simulink model "PUMA560robot_simulink"  (R2023a)
settings: Solver=ode4  StartTime=0.0  StopTime=10  FixedStep=0.001  RelTol=1e-3
values from neighbouring files (symbols this model uses):
  A = [zeros(3,3),eye(3,3) ... (first row only)    [main_PUMA560robot.m]
  B = [0   0   0 ... (first row only)    [main_PUMA560robot.m]
  d = norm(ep_-R_)    [main_PUMA560robot.m]
  Fcdirec = [1,100,1,0.001,           0.5,100,1,0.001,           1,300,1,0.3,           1,200,1,0.1,           2.5,100,2,0.01,           0.5,200,1,0.02]    [main_PUMA560robot.m]
  Kall = cat(1,Kall,K_)    [main_PUMA560robot.m]
  m = size(B',1)    [main_PUMA560robot.m]
  nK0 = 1    [main_PUMA560robot.m]
  Pall = cat(1,Pall,P_)    [main_PUMA560robot.m]
  R0q = Rall(1:3,1:3)    [main_PUMA560robot.m]
  rho = zeros(N,1)    [main_PUMA560robot.m]
  rhospan = linspace(0,1043,100000)    [main_PUMA560robot.m]
  umax = [97.8 136.4 89.4]    [main_PUMA560robot.m]
  x0 = 10/sqrt(6)* [1;1;1;1;1;1]    [main_PUMA560robot.m]
undefined symbols (not defined in the file or in its folder): Kb, Pb, Pcq
settings Model: Creator=shuyuanfan  LastModifiedBy=fansh

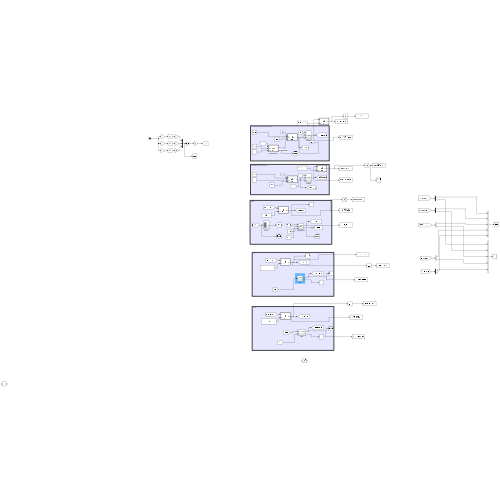
[thumbnail: Simulink's stored preview of the top-level diagram]
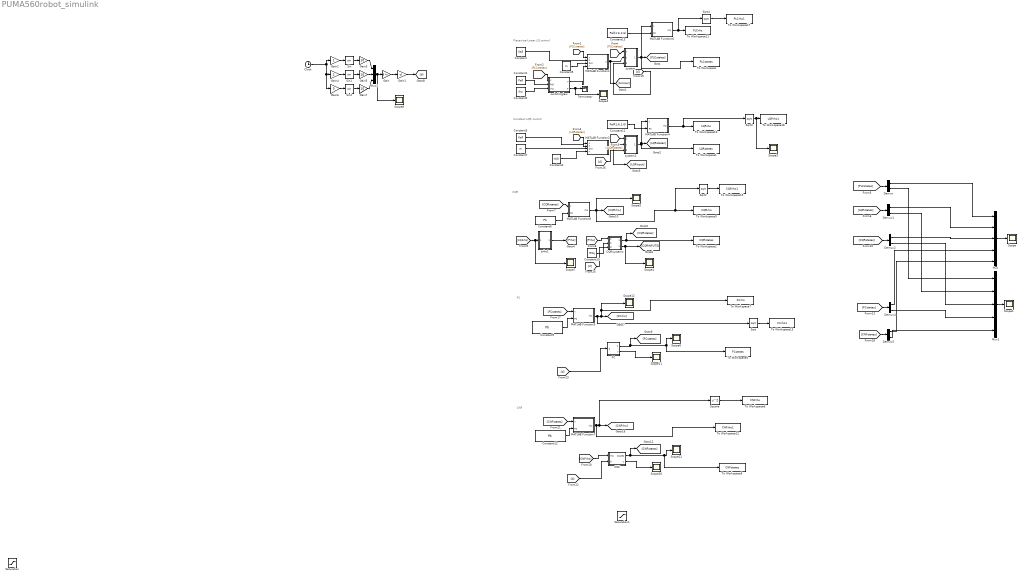
== system PUMA560robot_simulink ==
  note: CQR
  note: Piecewise-Linear LQ control
  note: Constant LQR control
  note: FC
  note: CNF
  CNF : Subsystem
  CQRsystems : Subsystem
  Clock : Clock
  Constant : Constant  Value=Kall
  Constant1 : Constant  Value=Pall
  Constant10 : Constant  Value=R0q
  Constant11 : Constant  Value=Pall(1:6,1:6)
  Constant12 : Constant  Value=Pb
  Constant13 : Constant  Value=Pall(1:6,1:6)
  Constant2 : Constant  Value=rho
  Constant3 : Constant  Value=Kall
  Constant4 : Constant  Value=nK0
  Constant5 : Constant  Value=m
  Constant6 : Constant  Value=Pb
  Constant7 : Constant  Value=m
  Constant9 : Constant  Value=Pb
  Demux{,1..2,4..5} (5 alike) : Demux  Outputs=2
  FC : Subsystem
  Gain : Gain  Gain=B  Multiplication=Matrix(K*u)
  Gain1 : Gain  Gain=d
  Gain2 : Gain
  Gain3 : Gain  Gain=10
  Gain4 : Gain  Gain=2
  Gain5 : Gain  Gain=10
  Gain6 : Gain  Gain=3
  Gain7 : Gain  Gain=10
  MATLAB Function1 : MATLAB Function  TreatAsAtomicUnit=on
  MATLAB Function2 : MATLAB Function  TreatAsAtomicUnit=on
  MATLAB Function3 : MATLAB Function  TreatAsAtomicUnit=on
  MATLAB Function4 : MATLAB Function  TreatAsAtomicUnit=on
  MATLAB Function6 : MATLAB Function  TreatAsAtomicUnit=on
  MATLAB Function7 : MATLAB Function  TreatAsAtomicUnit=on
  MATLAB Function8 : MATLAB Function  TreatAsAtomicUnit=on
  Mux : Mux  Inputs=5
  Mux1 : Mux  Inputs=5
  Mux2 : Mux  Inputs=3
  Saturation : Saturate  UpperLimit=umax'  LowerLimit=-umax'
  Saturation1 : Saturate  UpperLimit=umax'  LowerLimit=-umax'
  Scope{,1..8,11..12,20,22} (13 alike) : Scope
  Sin : Trigonometry
  Sin1 : Trigonometry
  Sin2 : Trigonometry
  Sqrt{,2..4} (4 alike) : Sqrt
  Square : Math  Operator=square
  Terminator : Terminator
  To Workspace : ToWorkspace  VariableName=PLCstates  SaveFormat=Timeseries  SampleTime=-1
  To Workspace1 : ToWorkspace  VariableName=LQRstates  SaveFormat=Timeseries  SampleTime=-1
  To Workspace10 : ToWorkspace  VariableName=LQRrho  SaveFormat=Timeseries  SampleTime=-1
  To Workspace11 : ToWorkspace  VariableName=PLCrho  SaveFormat=Timeseries  SampleTime=-1
  To Workspace12 : ToWorkspace  VariableName=CNFrho1  SaveFormat=Timeseries  SampleTime=-1
  To Workspace13 : ToWorkspace  VariableName=FCrho1  SaveFormat=Timeseries  SampleTime=-1
  To Workspace15 : ToWorkspace  VariableName=CQRrho1  SaveFormat=Timeseries  SampleTime=-1
  To Workspace16 : ToWorkspace  VariableName=LQRrho1  SaveFormat=Timeseries  SampleTime=-1
  To Workspace17 : ToWorkspace  VariableName=PLCrho1  SaveFormat=Timeseries  SampleTime=-1
  To Workspace2 : ToWorkspace  VariableName=CQRstates  SaveFormat=Timeseries  SampleTime=-1
  To Workspace4 : ToWorkspace  VariableName=FCstates  SaveFormat=Timeseries  SampleTime=-1
  To Workspace5 : ToWorkspace  VariableName=CNFstates  SaveFormat=Timeseries  SampleTime=-1
  To Workspace6 : ToWorkspace  VariableName=CNFrho  SaveFormat=Timeseries  SampleTime=-1
  To Workspace7 : ToWorkspace  VariableName=FCrho  SaveFormat=Timeseries  SampleTime=-1
  To Workspace9 : ToWorkspace  VariableName=CQRrho  SaveFormat=Timeseries  SampleTime=-1
  prho1 : Subsystem
  switchinglaw : MATLAB Function  TreatAsAtomicUnit=on
  system : Subsystem
  system2 : Subsystem
  wires:
  Constant/1 -> MATLAB Function1/2(K)
  Constant1/1 -> switchinglaw/2(Pall)
  Constant2/1 -> switchinglaw/3(rho)
  system/1(states) -> MATLAB Function6/1(x), To Workspace/1, [PLCstates]
  [PLCstates] -> system/1(x)
  [PLCstates] -> MATLAB Function1/1(x)
  [PLCstates] -> switchinglaw/1(x)
  MATLAB Function1/1(u) -> system/2(u), [PLCinput]
  MATLAB Function2/1(u) -> system2/2(u), [LQRinput]
  Constant3/1 -> MATLAB Function2/2(K)
  Constant4/1 -> MATLAB Function2/4(n)
  system2/1(states) -> MATLAB Function4/1(x), [LQRstates], To Workspace1/1
  [LQRstates] -> MATLAB Function2/1(x)
  Constant7/1 -> MATLAB Function2/3(dim)
  [LQRstates] -> system2/1(x)
  switchinglaw/1(n) -> MATLAB Function1/4(n)
  Constant5/1 -> MATLAB Function1/3(dim)
  switchinglaw/2(F) -> Scope2/1, Terminator/1
  [CQRstates] -> MATLAB Function8/1(x)
  [CQRrho] -> Scope7/1, prho1/1(In1)
  MATLAB Function8/1(rho) -> Scope5/1, Sqrt2/1, To Workspace9/1, [CQRrho]
  Constant6/1 -> MATLAB Function8/2(P0)
  CQRsystems/2(u) -> Scope4/1, [CQRINPUTS]
  CQRsystems/1(states) -> To Workspace2/1, [CQRstates]
  [Prho] -> CQRsystems/1(p)
  Constant10/1 -> CQRsystems/2(paraR)
  prho1/1(Out1) -> [Prho]
  FC/2(u) -> Scope11/1
  FC/1(states) -> Scope6/1, To Workspace4/1, [FCstates]
  [FCstates] -> MATLAB Function3/1(x)
  Constant9/1 -> MATLAB Function3/2(P0)
  MATLAB Function3/1(rho) -> Sqrt/1, To Workspace7/1, Scope12/1, [FCrho]
  [CNFstates] -> MATLAB Function7/1(x)
  CNF/2(u) -> Scope20/1
  [CNFrho] -> CNF/1(rho)
  Constant12/1 -> MATLAB Function7/2(P0)
  MATLAB Function7/1(rho) -> To Workspace12/1, Square/1, [CNFrho]
  CNF/1(states) -> To Workspace5/1, Scope22/1, [CNFstates]
  [PLCstates] -> Demux/1
  [LQRstates] -> Demux1/1
  [CQRstates] -> Demux2/1
  [FCstates] -> Demux4/1
  [CNFstates] -> Demux5/1
  Demux/1 -> Mux/1
  Demux1/1 -> Mux/2
  Demux2/1 -> Mux/3
  Demux4/1 -> Mux/4
  Demux5/1 -> Mux/5
  Demux/2 -> Mux1/1
  Demux1/2 -> Mux1/2
  Demux2/2 -> Mux1/3
  Demux4/2 -> Mux1/4
  Demux5/2 -> Mux1/5
  Mux/1 -> Scope/1
  Mux1/1 -> Scope1/1
  Square/1 -> To Workspace6/1
  MATLAB Function4/1(rho) -> Sqrt3/1, To Workspace10/1
  Constant11/1 -> MATLAB Function4/2(P0)
  Constant13/1 -> MATLAB Function6/2(P0)
  MATLAB Function6/1(rho) -> Sqrt4/1, To Workspace11/1
  Sqrt/1 -> To Workspace13/1
  Sqrt2/1 -> To Workspace15/1
  Sqrt3/1 -> Scope3/1, To Workspace16/1
  Sqrt4/1 -> To Workspace17/1
  Gain1/1 -> [d]
  [d] -> system/3(d)
  [d] -> system2/3(d)
  [d] -> CQRsystems/3(d)
  [d] -> FC/1(d)
  [d] -> CNF/2(d)
  Gain/1 -> Gain1/1
  Gain2/1 -> Sin/1
  Sin/1 -> Gain3/1
  Sin1/1 -> Gain5/1
  Gain4/1 -> Sin1/1
  Clock/1 -> Gain6/1, Gain4/1, Gain2/1
  Sin2/1 -> Gain7/1
  Gain6/1 -> Sin2/1
  Gain5/1 -> Mux2/2
  Gain3/1 -> Mux2/1
  Gain7/1 -> Mux2/3
  Mux2/1 -> Scope8/1, Gain/1

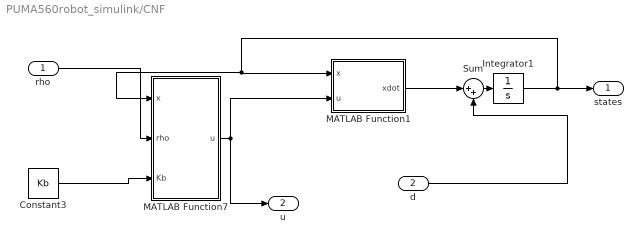
== system PUMA560robot_simulink/CNF ==
  rho : Inport
  d : Inport  Port=2
  Constant3 : Constant  Value=Kb
  Integrator1 : Integrator  InitialCondition=x0
  MATLAB Function1 : MATLAB Function  TreatAsAtomicUnit=on
  MATLAB Function7 : MATLAB Function  TreatAsAtomicUnit=on
  Sum : Sum  Inputs=|++
  states : Outport
  u : Outport  Port=2
  wires:
  Integrator1/1 -> states/1, MATLAB Function1/1(x), MATLAB Function7/1(x)
  MATLAB Function1/1(xdot) -> Sum/1
  Sum/1 -> Integrator1/1
  d/1 -> Sum/2
  rho/1 -> MATLAB Function7/2(rho)
  Constant3/1 -> MATLAB Function7/3(Kb)
  MATLAB Function7/1(u) -> MATLAB Function1/2(u), u/1

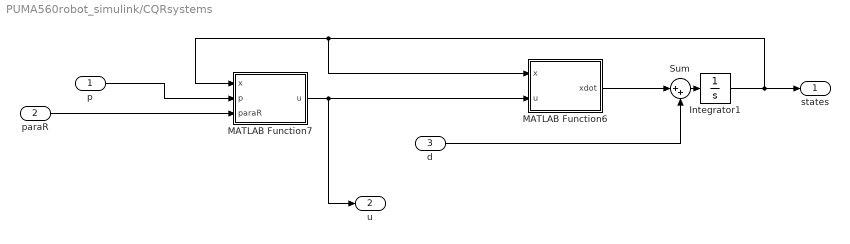
== system PUMA560robot_simulink/CQRsystems ==
  p : Inport
  paraR : Inport  Port=2
  d : Inport  Port=3
  Integrator1 : Integrator  InitialCondition=x0
  MATLAB Function6 : MATLAB Function  TreatAsAtomicUnit=on
  MATLAB Function7 : MATLAB Function  TreatAsAtomicUnit=on
  Sum : Sum  Inputs=|++
  states : Outport
  u : Outport  Port=2
  wires:
  Integrator1/1 -> states/1, MATLAB Function6/1(x), MATLAB Function7/1(x)
  MATLAB Function6/1(xdot) -> Sum/1
  paraR/1 -> MATLAB Function7/3(paraR)
  p/1 -> MATLAB Function7/2(p)
  Sum/1 -> Integrator1/1
  d/1 -> Sum/2
  MATLAB Function7/1(u) -> MATLAB Function6/2(u), u/1

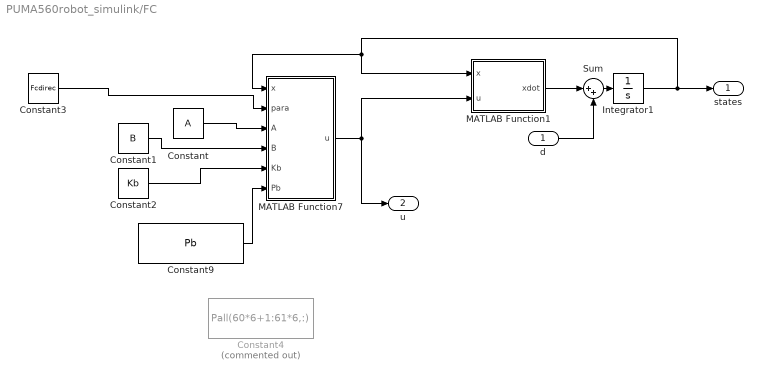
== system PUMA560robot_simulink/FC ==
  d : Inport
  Constant : Constant  Value=A
  Constant1 : Constant  Value=B
  Constant2 : Constant  Value=Kb
  Constant3 : Constant  Value=Fcdirec
  Constant4 : Constant  Commented=on  Value=Pall(60*6+1:61*6,:)
  Constant9 : Constant  Value=Pb
  Integrator1 : Integrator  InitialCondition=x0
  MATLAB Function1 : MATLAB Function  TreatAsAtomicUnit=on
  MATLAB Function7 : MATLAB Function  TreatAsAtomicUnit=on
  Sum : Sum  Inputs=|++
  states : Outport
  u : Outport  Port=2
  wires:
  Integrator1/1 -> states/1, MATLAB Function1/1(x), MATLAB Function7/1(x)
  MATLAB Function1/1(xdot) -> Sum/1
  Sum/1 -> Integrator1/1
  Constant/1 -> MATLAB Function7/3(A)
  Constant1/1 -> MATLAB Function7/4(B)
  Constant2/1 -> MATLAB Function7/5(Kb)
  Constant9/1 -> MATLAB Function7/6(Pb)
  d/1 -> Sum/2
  MATLAB Function7/1(u) -> MATLAB Function1/2(u), u/1
  Constant3/1 -> MATLAB Function7/2(para)

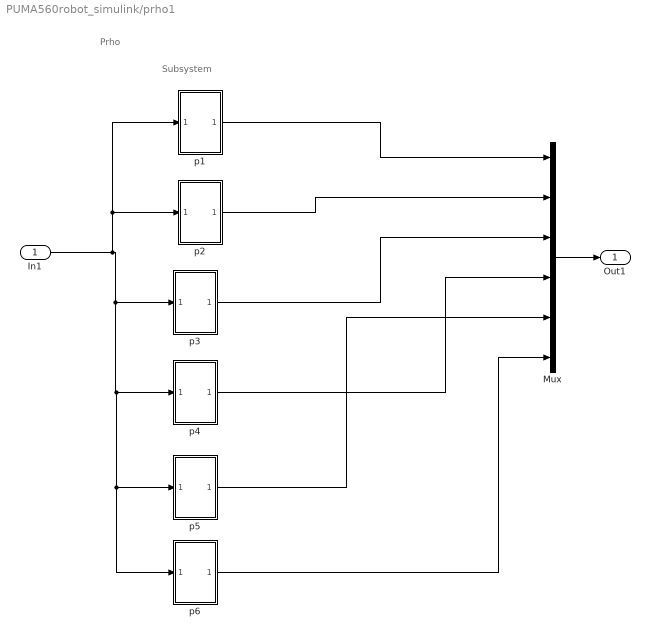
== system PUMA560robot_simulink/prho1 ==
  note: Prho
  note: Subsystem
  In1 : Inport
  Mux : Mux  Inputs=6
  p1 : Subsystem
  p2 : Subsystem
  p3 : Subsystem
  p4 : Subsystem
  p5 : Subsystem
  p6 : Subsystem
  Out1 : Outport
  wires:
  p4/1(Out1) -> Mux/4
  In1/1 -> p6/1(In1), p5/1(In1), p4/1(In1), p3/1(In1), p2/1(In1), p1/1(In1)
  Mux/1 -> Out1/1
  p1/1(Out1) -> Mux/1
  p3/1(Out1) -> Mux/3
  p2/1(Out1) -> Mux/2
  p5/1(Out1) -> Mux/5
  p6/1(Out1) -> Mux/6

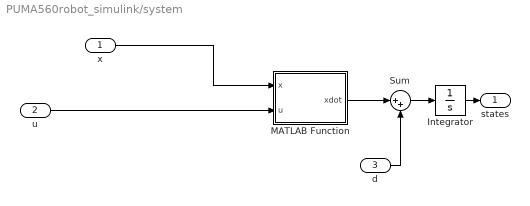
== system PUMA560robot_simulink/system ==
  x : Inport
  u : Inport  Port=2
  d : Inport  Port=3
  Integrator : Integrator  InitialCondition=x0
  MATLAB Function : MATLAB Function  TreatAsAtomicUnit=on
  Sum : Sum  Inputs=|++
  states : Outport
  wires:
  x/1 -> MATLAB Function/1(x)
  Integrator/1 -> states/1
  MATLAB Function/1(xdot) -> Sum/1
  Sum/1 -> Integrator/1
  d/1 -> Sum/2
  u/1 -> MATLAB Function/2(u)

== system PUMA560robot_simulink/system2 ==
  x : Inport
  u : Inport  Port=2
  d : Inport  Port=3
  Integrator : Integrator  InitialCondition=x0
  MATLAB Function : MATLAB Function  TreatAsAtomicUnit=on
  Sum : Sum  Inputs=|++
  states : Outport
  wires:
  x/1 -> MATLAB Function/1(x)
  Integrator/1 -> states/1
  MATLAB Function/1(xdot) -> Sum/1
  Sum/1 -> Integrator/1
  d/1 -> Sum/2
  u/1 -> MATLAB Function/2(u)

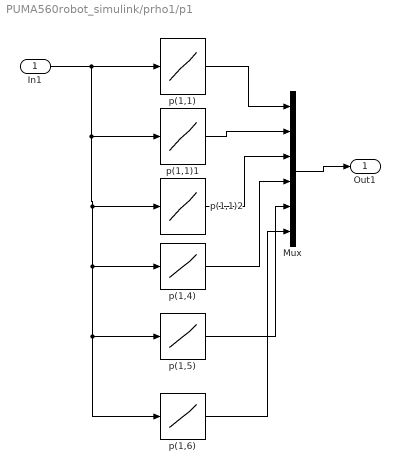
== system PUMA560robot_simulink/prho1/p1 ==
  In1 : Inport
  Mux : Mux  Inputs=6
  p(1,1) : Lookup_n-D  NumberOfTableDimensions=1  BreakpointsForDimension1=rhospan  Table=Pcq(:,1)  InterpMethod=Linear Lagrange  InternalRulePriority=Speed  RndMeth=Simplest
  p(1,1)1 : Lookup_n-D  NumberOfTableDimensions=1  BreakpointsForDimension1=rhospan  Table=Pcq(:,2)  InterpMethod=Linear Lagrange  InternalRulePriority=Speed  RndMeth=Simplest
  p(1,1)2 : Lookup_n-D  NumberOfTableDimensions=1  BreakpointsForDimension1=rhospan  Table=Pcq(:,3)  InterpMethod=Linear Lagrange  InternalRulePriority=Speed  RndMeth=Simplest
  p(1,4) : Lookup_n-D  NumberOfTableDimensions=1  BreakpointsForDimension1=rhospan  Table=Pcq(:,4)  InterpMethod=Linear Lagrange  InternalRulePriority=Speed  RndMeth=Simplest
  p(1,5) : Lookup_n-D  NumberOfTableDimensions=1  BreakpointsForDimension1=rhospan  Table=Pcq(:,5)  InterpMethod=Linear Lagrange  InternalRulePriority=Speed  RndMeth=Simplest
  p(1,6) : Lookup_n-D  NumberOfTableDimensions=1  BreakpointsForDimension1=rhospan  Table=Pcq(:,6)  InterpMethod=Linear Lagrange  InternalRulePriority=Speed  RndMeth=Simplest
  Out1 : Outport
  wires:
  p(1,1)1/1 -> Mux/2
  p(1,4)/1 -> Mux/4
  In1/1 -> p(1,1)1/1, p(1,1)2/1, p(1,6)/1, p(1,5)/1, p(1,4)/1, p(1,1)/1
  p(1,1)/1 -> Mux/1
  p(1,1)2/1 -> Mux/3
  Mux/1 -> Out1/1
  p(1,5)/1 -> Mux/5
  p(1,6)/1 -> Mux/6

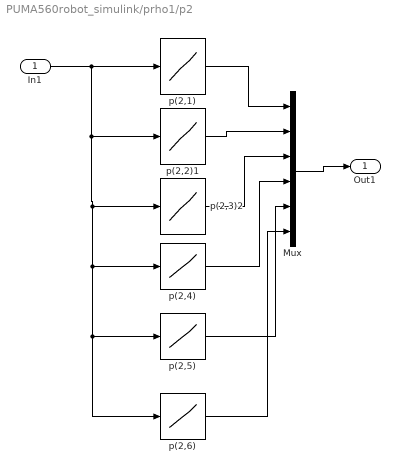
== system PUMA560robot_simulink/prho1/p2 ==
  In1 : Inport
  Mux : Mux  Inputs=6
  p(2,1) : Lookup_n-D  NumberOfTableDimensions=1  BreakpointsForDimension1=rhospan  Table=Pcq(:,7)  InterpMethod=Linear Lagrange  InternalRulePriority=Speed  RndMeth=Simplest
  p(2,2)1 : Lookup_n-D  NumberOfTableDimensions=1  BreakpointsForDimension1=rhospan  Table=Pcq(:,8)  InterpMethod=Linear Lagrange  InternalRulePriority=Speed  RndMeth=Simplest
  p(2,3)2 : Lookup_n-D  NumberOfTableDimensions=1  BreakpointsForDimension1=rhospan  Table=Pcq(:,9)  InterpMethod=Linear Lagrange  InternalRulePriority=Speed  RndMeth=Simplest
  p(2,4) : Lookup_n-D  NumberOfTableDimensions=1  BreakpointsForDimension1=rhospan  Table=Pcq(:,10)  InterpMethod=Linear Lagrange  InternalRulePriority=Speed  RndMeth=Simplest
  p(2,5) : Lookup_n-D  NumberOfTableDimensions=1  BreakpointsForDimension1=rhospan  Table=Pcq(:,11)  InterpMethod=Linear Lagrange  InternalRulePriority=Speed  RndMeth=Simplest
  p(2,6) : Lookup_n-D  NumberOfTableDimensions=1  BreakpointsForDimension1=rhospan  Table=Pcq(:,12)  InterpMethod=Linear Lagrange  InternalRulePriority=Speed  RndMeth=Simplest
  Out1 : Outport
  wires:
  p(2,2)1/1 -> Mux/2
  p(2,4)/1 -> Mux/4
  In1/1 -> p(2,2)1/1, p(2,3)2/1, p(2,6)/1, p(2,5)/1, p(2,4)/1, p(2,1)/1
  p(2,1)/1 -> Mux/1
  p(2,3)2/1 -> Mux/3
  Mux/1 -> Out1/1
  p(2,5)/1 -> Mux/5
  p(2,6)/1 -> Mux/6

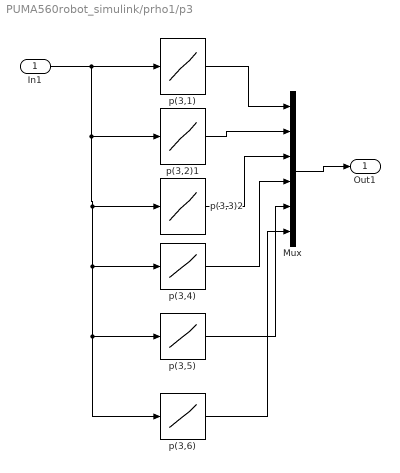
== system PUMA560robot_simulink/prho1/p3 ==
  In1 : Inport
  Mux : Mux  Inputs=6
  p(3,1) : Lookup_n-D  NumberOfTableDimensions=1  BreakpointsForDimension1=rhospan  Table=Pcq(:,13)  InterpMethod=Linear Lagrange  InternalRulePriority=Speed  RndMeth=Simplest
  p(3,2)1 : Lookup_n-D  NumberOfTableDimensions=1  BreakpointsForDimension1=rhospan  Table=Pcq(:,14)  InterpMethod=Linear Lagrange  InternalRulePriority=Speed  RndMeth=Simplest
  p(3,3)2 : Lookup_n-D  NumberOfTableDimensions=1  BreakpointsForDimension1=rhospan  Table=Pcq(:,15)  InterpMethod=Linear Lagrange  InternalRulePriority=Speed  RndMeth=Simplest
  p(3,4) : Lookup_n-D  NumberOfTableDimensions=1  BreakpointsForDimension1=rhospan  Table=Pcq(:,16)  InterpMethod=Linear Lagrange  InternalRulePriority=Speed  RndMeth=Simplest
  p(3,5) : Lookup_n-D  NumberOfTableDimensions=1  BreakpointsForDimension1=rhospan  Table=Pcq(:,17)  InterpMethod=Linear Lagrange  InternalRulePriority=Speed  RndMeth=Simplest
  p(3,6) : Lookup_n-D  NumberOfTableDimensions=1  BreakpointsForDimension1=rhospan  Table=Pcq(:,18)  InterpMethod=Linear Lagrange  InternalRulePriority=Speed  RndMeth=Simplest
  Out1 : Outport
  wires:
  p(3,2)1/1 -> Mux/2
  p(3,4)/1 -> Mux/4
  In1/1 -> p(3,2)1/1, p(3,3)2/1, p(3,6)/1, p(3,5)/1, p(3,4)/1, p(3,1)/1
  p(3,1)/1 -> Mux/1
  p(3,3)2/1 -> Mux/3
  Mux/1 -> Out1/1
  p(3,5)/1 -> Mux/5
  p(3,6)/1 -> Mux/6

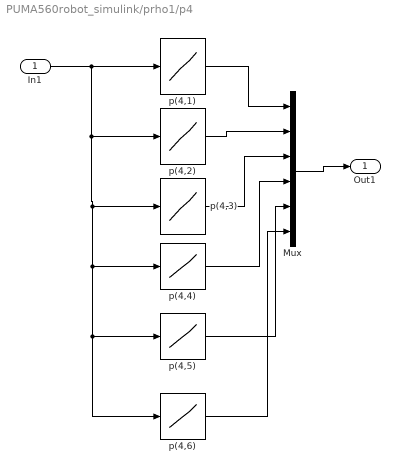
== system PUMA560robot_simulink/prho1/p4 ==
  In1 : Inport
  Mux : Mux  Inputs=6
  p(4,1) : Lookup_n-D  NumberOfTableDimensions=1  BreakpointsForDimension1=rhospan  Table=Pcq(:,19)  InterpMethod=Linear Lagrange  InternalRulePriority=Speed  RndMeth=Simplest
  p(4,2) : Lookup_n-D  NumberOfTableDimensions=1  BreakpointsForDimension1=rhospan  Table=Pcq(:,20)  InterpMethod=Linear Lagrange  InternalRulePriority=Speed  RndMeth=Simplest
  p(4,3) : Lookup_n-D  NumberOfTableDimensions=1  BreakpointsForDimension1=rhospan  Table=Pcq(:,21)  InterpMethod=Linear Lagrange  InternalRulePriority=Speed  RndMeth=Simplest
  p(4,4) : Lookup_n-D  NumberOfTableDimensions=1  BreakpointsForDimension1=rhospan  Table=Pcq(:,22)  InterpMethod=Linear Lagrange  InternalRulePriority=Speed  RndMeth=Simplest
  p(4,5) : Lookup_n-D  NumberOfTableDimensions=1  BreakpointsForDimension1=rhospan  Table=Pcq(:,23)  InterpMethod=Linear Lagrange  InternalRulePriority=Speed  RndMeth=Simplest
  p(4,6) : Lookup_n-D  NumberOfTableDimensions=1  BreakpointsForDimension1=rhospan  Table=Pcq(:,24)  InterpMethod=Linear Lagrange  InternalRulePriority=Speed  RndMeth=Simplest
  Out1 : Outport
  wires:
  p(4,2)/1 -> Mux/2
  p(4,4)/1 -> Mux/4
  In1/1 -> p(4,2)/1, p(4,3)/1, p(4,6)/1, p(4,5)/1, p(4,4)/1, p(4,1)/1
  p(4,1)/1 -> Mux/1
  p(4,3)/1 -> Mux/3
  Mux/1 -> Out1/1
  p(4,5)/1 -> Mux/5
  p(4,6)/1 -> Mux/6

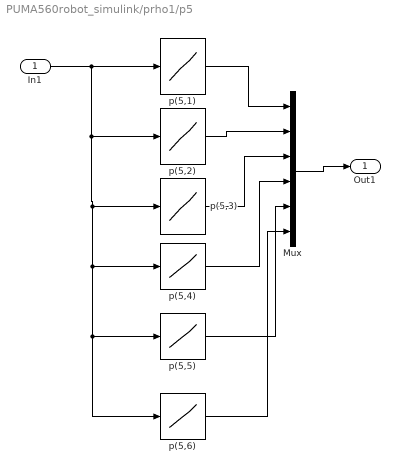
== system PUMA560robot_simulink/prho1/p5 ==
  In1 : Inport
  Mux : Mux  Inputs=6
  p(5,1) : Lookup_n-D  NumberOfTableDimensions=1  BreakpointsForDimension1=rhospan  Table=Pcq(:,25)  InterpMethod=Linear Lagrange  InternalRulePriority=Speed  RndMeth=Simplest
  p(5,2) : Lookup_n-D  NumberOfTableDimensions=1  BreakpointsForDimension1=rhospan  Table=Pcq(:,26)  InterpMethod=Linear Lagrange  InternalRulePriority=Speed  RndMeth=Simplest
  p(5,3) : Lookup_n-D  NumberOfTableDimensions=1  BreakpointsForDimension1=rhospan  Table=Pcq(:,27)  InterpMethod=Linear Lagrange  InternalRulePriority=Speed  RndMeth=Simplest
  p(5,4) : Lookup_n-D  NumberOfTableDimensions=1  BreakpointsForDimension1=rhospan  Table=Pcq(:,28)  InterpMethod=Linear Lagrange  InternalRulePriority=Speed  RndMeth=Simplest
  p(5,5) : Lookup_n-D  NumberOfTableDimensions=1  BreakpointsForDimension1=rhospan  Table=Pcq(:,29)  InterpMethod=Linear Lagrange  InternalRulePriority=Speed  RndMeth=Simplest
  p(5,6) : Lookup_n-D  NumberOfTableDimensions=1  BreakpointsForDimension1=rhospan  Table=Pcq(:,30)  InterpMethod=Linear Lagrange  InternalRulePriority=Speed  RndMeth=Simplest
  Out1 : Outport
  wires:
  p(5,2)/1 -> Mux/2
  p(5,4)/1 -> Mux/4
  In1/1 -> p(5,2)/1, p(5,3)/1, p(5,6)/1, p(5,5)/1, p(5,4)/1, p(5,1)/1
  p(5,1)/1 -> Mux/1
  p(5,3)/1 -> Mux/3
  Mux/1 -> Out1/1
  p(5,5)/1 -> Mux/5
  p(5,6)/1 -> Mux/6

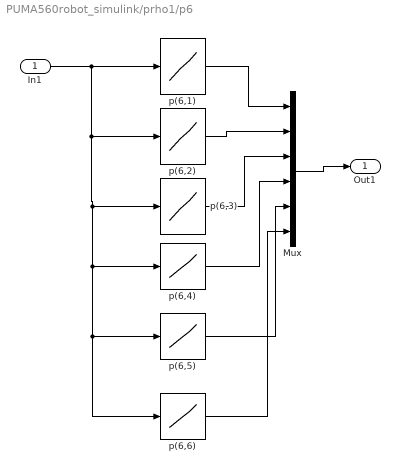
== system PUMA560robot_simulink/prho1/p6 ==
  In1 : Inport
  Mux : Mux  Inputs=6
  p(6,1) : Lookup_n-D  NumberOfTableDimensions=1  BreakpointsForDimension1=rhospan  Table=Pcq(:,31)  InterpMethod=Linear Lagrange  InternalRulePriority=Speed  RndMeth=Simplest
  p(6,2) : Lookup_n-D  NumberOfTableDimensions=1  BreakpointsForDimension1=rhospan  Table=Pcq(:,32)  InterpMethod=Linear Lagrange  InternalRulePriority=Speed  RndMeth=Simplest
  p(6,3) : Lookup_n-D  NumberOfTableDimensions=1  BreakpointsForDimension1=rhospan  Table=Pcq(:,33)  InterpMethod=Linear Lagrange  InternalRulePriority=Speed  RndMeth=Simplest
  p(6,4) : Lookup_n-D  NumberOfTableDimensions=1  BreakpointsForDimension1=rhospan  Table=Pcq(:,34)  InterpMethod=Linear Lagrange  InternalRulePriority=Speed  RndMeth=Simplest
  p(6,5) : Lookup_n-D  NumberOfTableDimensions=1  BreakpointsForDimension1=rhospan  Table=Pcq(:,35)  InterpMethod=Linear Lagrange  InternalRulePriority=Speed  RndMeth=Simplest
  p(6,6) : Lookup_n-D  NumberOfTableDimensions=1  BreakpointsForDimension1=rhospan  Table=Pcq(:,36)  InterpMethod=Linear Lagrange  InternalRulePriority=Speed  RndMeth=Simplest
  Out1 : Outport
  wires:
  p(6,2)/1 -> Mux/2
  p(6,4)/1 -> Mux/4
  In1/1 -> p(6,2)/1, p(6,3)/1, p(6,6)/1, p(6,5)/1, p(6,4)/1, p(6,1)/1
  p(6,1)/1 -> Mux/1
  p(6,3)/1 -> Mux/3
  Mux/1 -> Out1/1
  p(6,5)/1 -> Mux/5
  p(6,6)/1 -> Mux/6

== matlab function PUMA560robot_simulink/MATLAB Function4 ==
  data: x input; rho output; P0 input
function rho = fcn(x,P0)

rho = x'*P0*x;

== matlab function PUMA560robot_simulink/MATLAB Function6 ==
  data: x input; rho output; P0 input
function rho = fcn(x,P0)

rho = x'*P0*x;

== matlab function PUMA560robot_simulink/system2/MATLAB Function ==
  data: x input; u input; xdot output
function xdot= fcn(x,u)
%A = [0 1; -10 0];
%B = [0;1];
A = [zeros(3,3),eye(3,3);
    0 -0.0451 -0.0451 0 0 0;
    0 -0.0457 -0.0457 0 0 0;
    0 -4.5551 -4.5551 0 0 0];

B = [0   0   0;
     0   0   0;
     0   0   0;
     0.0925 0 0.0026;
     0    0.0979  -0.0952;
     0.0026  -0.0954  0.3616];

xdot = A*x+B*u;

== matlab function PUMA560robot_simulink/CNF/MATLAB Function1 ==
  data: x input; u input; xdot output
function xdot= fcn(x,u)
%A = [0 1; -10 0];
%B = [0;1];
A = [zeros(3,3),eye(3,3);
    0 -0.0451 -0.0451 0 0 0;
    0 -0.0457 -0.0457 0 0 0;
    0 -4.5551 -4.5551 0 0 0];

B = [0   0   0;
     0   0   0;
     0   0   0;
     0.0925 0 0.0026;
     0    0.0979  -0.0952;
     0.0026  -0.0954  0.3616];

xdot = A*x+B*u;

== matlab function PUMA560robot_simulink/CNF/MATLAB Function7 ==
  data: x input; u output; rho input; Kb input
function u= fcn(x,rho,Kb)

%[T,~] = eig(Mb);
K =Kb+200* exp(-0.65*rho)*Kb;
%K = Kb;

u =- K*x;

== matlab function PUMA560robot_simulink/MATLAB Function7 ==
  data: x input; rho output; P0 input
function rho = fcn(x,P0)

%rho = x'*P0*x;

rho = sqrt(x'*P0*x);

== matlab function PUMA560robot_simulink/MATLAB Function1 ==
  data: x input; u output; K input; dim input; n input
function u = fcn(x,K,dim,n)
udim = dim;
%selector = n*dim-2;
%Kuse = zeros(dim,6);
%Kuse(1,:)=K(n*dim-2,:);
%Kuse(2,:)=K(n*dim-1,:);
%Kuse(3,:)=K(n*dim,:);
%Kuse = K(selector:n*dim,1:6);
%u = zeros(3,1);
%u(1) = -Kuse(1,:)*x;
%u(2) = -Kuse(2,:)*x;
%u(3) = -Kuse(3,:)*x;
d = -K((n*udim-udim+1):(n*udim),:)*x;
u = zeros(3,1);
u(1)=d(1);
u(2)=d(2);
u(3)=d(3);
end

== matlab function PUMA560robot_simulink/system/MATLAB Function ==
  data: x input; u input; xdot output
function xdot= fcn(x,u)
%A = [0 1; -10 0];
%B = [0;1];
A = [zeros(3,3),eye(3,3);
    0 -0.0451 -0.0451 0 0 0;
    0 -0.0457 -0.0457 0 0 0;
    0 -4.5551 -4.5551 0 0 0];

B = [0   0   0;
     0   0   0;
     0   0   0;
     0.0925 0 0.0026;
     0    0.0979  -0.0952;
     0.0026  -0.0954  0.3616];

xdot = A*x+B*u;

== matlab function PUMA560robot_simulink/switchinglaw ==
  data: x input; n output; Pall input; rho input; F output
function [n,F] = fcn(x,Pall,rho)
N = size(rho,1);
i = 1;
xdim = size(Pall',1);
%udim = dim;
F = zeros(N,1);
for i = 1:N
    P = Pall(i*xdim-xdim+1:i*xdim,:);
    F(i) = sign(rho(i)-x'*P*x);
end
n=1;
for i = 1:N-1
    d = F(i)*F(i+1);
    if d<0
        n = i;
    end
end

if F(1)*F(N)>0&&F(1)>0
    n = N;
end
if F(1)*F(N)>0&&F(1)<0
    n = 1;
end

== matlab function PUMA560robot_simulink/MATLAB Function2 ==
  data: x input; u output; K input; dim input; n input
function u = fcn(x,K,dim,n)
udim = 3;
u = zeros(udim,1);
Kuse = K(n*udim-udim+1:n*udim,:);
d = -Kuse*x ;
u(1)=d(1);
u(2)=d(2);
u(3)=d(3);
end

== matlab function PUMA560robot_simulink/CQRsystems/MATLAB Function6 ==
  data: x input; u input; xdot output
function xdot= fcn(x,u)
%A = [0 1; -10 0];
%B = [0;1];
A = [zeros(3,3),eye(3,3);
    0 -0.0451 -0.0451 0 0 0;
    0 -0.0457 -0.0457 0 0 0;
    0 -4.5551 -4.5551 0 0 0];

B = [0   0   0;
     0   0   0;
     0   0   0;
     0.0925 0 0.0026;
     0    0.0979  -0.0952;
     0.0026  -0.0954  0.3616];

xdot = A*x+B*u;

== matlab function PUMA560robot_simulink/FC/MATLAB Function1 ==
  data: x input; u input; xdot output
function xdot= fcn(x,u)
%A = [0 1; -10 0];
%B = [0;1];
A = [zeros(3,3),eye(3,3);
    0 -0.0451 -0.0451 0 0 0;
    0 -0.0457 -0.0457 0 0 0;
    0 -4.5551 -4.5551 0 0 0];

B = [0   0   0;
     0   0   0;
     0   0   0;
     0.0925 0 0.0026;
     0    0.0979  -0.0952;
     0.0026  -0.0954  0.3616];

xdot = A*x+B*u;

== matlab function PUMA560robot_simulink/CQRsystems/MATLAB Function7 ==
  data: x input; u output; p input; paraR input
function u= fcn(x,p,paraR)
R =paraR;

% system matrix
A = [zeros(3,3),eye(3,3);
    0 -0.0451 -0.0451 0 0 0;
    0 -0.0457 -0.0457 0 0 0;
    0 -4.5551 -4.5551 0 0 0];

B = [0   0   0;
     0   0   0;
     0   0   0;
     0.0925 0 0.0026;
     0    0.0979  -0.0952;
     0.0026  -0.0954  0.3616];

p_ = reshape(p,[6,6]);
P = p_';
R_inv = inv(R);
u = -R_inv*B'*P*x;

== matlab function PUMA560robot_simulink/FC/MATLAB Function7 ==
  data: x input; u output; para input; A input; B input; Kb input; Pb input


function u = fcn(x,para,A,B,Kb,Pb)

%Concave factor
rho = x'*Pb*x;
rho = sqrt(rho);
f1 = fcs2(rho,para(1:4));
f2 = fcs2(rho,para(5:8));
f3 = fcs2(rho,para(9:12));
f4 = fcs2(rho,para(13:16));
f5 = fcs2(rho,para(17:20));
f6 = fcs2(rho,para(21:24));
Fc = diag([f1,f2,f3,f4,f5,f6]);

% compute baseline closed-loop matrix
Acl = A - B*Kb;

% baseline Mb
Mb = -(Acl'*Pb + Pb*Acl);


%Directly improve the eigenvalue of Pb
[Tb,~] = eig(Pb);
Tb = real(Tb);
Tb = inv(Tb);

Fcsqrt = sqrtm(Fc);
Fcsqrt = real(Fcsqrt);
Gam = inv(Tb)*Fcsqrt*Tb;

Kn = inv(B'*B)*B'*(A-Gam'*Acl*Gam');

u = -Kn*x;

end

== matlab function PUMA560robot_simulink/MATLAB Function8 ==
  data: x input; rho output; P0 input
function rho = fcn(x,P0)

rho = x'*P0*x;

== matlab function PUMA560robot_simulink/MATLAB Function3 ==
  data: x input; rho output; P0 input
function rho = fcn(x,P0)

rho = x'*P0*x;

%rho = sqrt(x'*P0*x);
